simulink model "thruster_dynamics_test"  (R2016a)
settings: Solver=VariableStepAuto  StartTime=0.0  StopTime=1000.0  RelTol=1e-3
undefined symbols (not defined in the file or in its folder): forces_and_moments, P
libraries: simulink x4
settings Model: Creator=drew  LastModifiedBy=andrew
settings DataIOCC: LimitDataPoints=on
settings DebuggingCC: AllowSymbolicDim=off
settings ModelReferenceCC: PropagateSignalLabelsOutOfModel=off
settings GRTTargetCC: GeneratePreprocessorConditionals=Use local settings

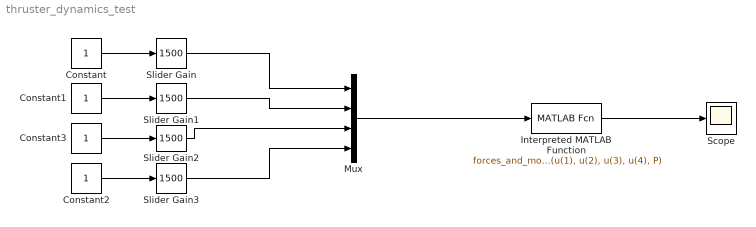
== system thruster_dynamics_test ==
  Constant{,1..3} (4 alike) : Constant
  Interpreted MATLAB Function : MATLABFcn  MATLABFcn=forces_and_moments(u(1), u(2), u(3), u(4), P)  OutputDimensions=6
  Mux : Mux
  Scope : Scope
  Slider Gain{,1..3} (4 alike) : simulink/Math Operations/Slider Gain  low=1100  gain=1500  high=1900
  wires:
  Slider Gain/1 -> Mux/1
  Slider Gain1/1 -> Mux/2
  Slider Gain2/1 -> Mux/3
  Slider Gain3/1 -> Mux/4
  Constant/1 -> Slider Gain/1
  Constant3/1 -> Slider Gain2/1
  Constant1/1 -> Slider Gain1/1
  Constant2/1 -> Slider Gain3/1
  Mux/1 -> Interpreted MATLAB Function/1
  Interpreted MATLAB Function/1 -> Scope/1
